simulink model "BatteryModel2RC"  (R2019a)
settings: Solver=VariableStepAuto  StartTime=0.0  StopTime=2417.4  RelTol=1e-3
undefined symbols (not defined in the file): C1Prime, C2Prime, CapacityAh, DiscIntNeverNeededParam, Em, R0, Rx, SOC_LUT
settings Model: Creator=danis  LastModifiedBy=danis

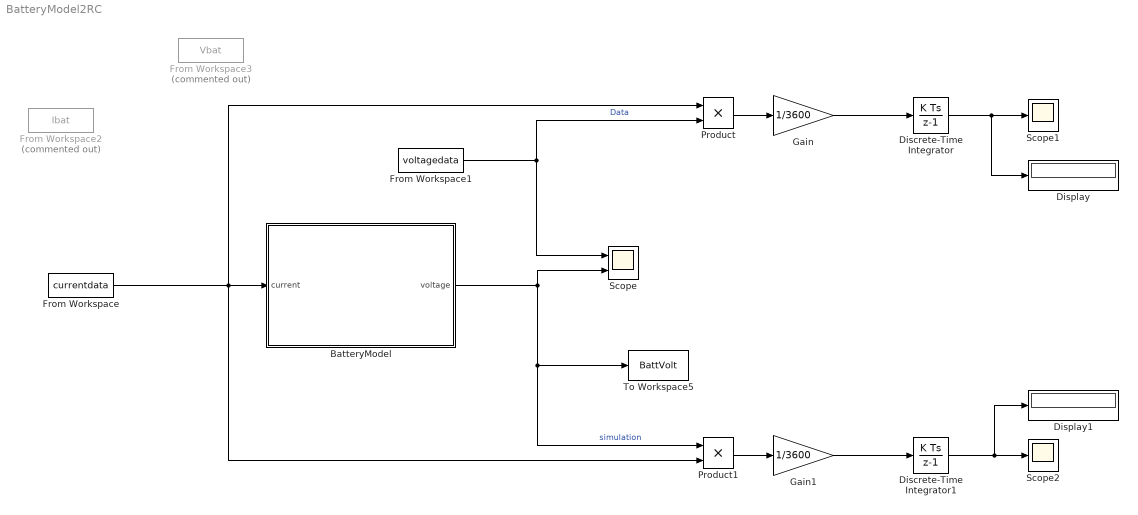
== system BatteryModel2RC ==
  BatteryModel : Subsystem
  Discrete-Time Integrator : DiscreteIntegrator  SampleTime=-1  ICPrevOutput=DiscIntNeverNeededParam  ICPrevScaledInput=DiscIntNeverNeededParam
  Discrete-Time Integrator1 : DiscreteIntegrator  SampleTime=-1  ICPrevOutput=DiscIntNeverNeededParam  ICPrevScaledInput=DiscIntNeverNeededParam
  Display : Display
  Display1 : Display
  From Workspace : FromWorkspace  VariableName=currentdata  SampleTime=0
  From Workspace1 : FromWorkspace  VariableName=voltagedata  SampleTime=0
  From Workspace2 : FromWorkspace  Commented=on  VariableName=Ibat  SampleTime=0.001  Interpolate=off  OutputAfterFinalValue=Cyclic repetition
  From Workspace3 : FromWorkspace  Commented=on  VariableName=Vbat  SampleTime=0.001  Interpolate=off  OutputAfterFinalValue=Cyclic repetition
  Gain : Gain  Gain=1/3600
  Gain1 : Gain  Gain=1/3600
  Product : Product
  Product1 : Product
  Scope : Scope  NumInputPorts=2
  Scope1 : Scope
  Scope2 : Scope
  To Workspace5 : ToWorkspace  VariableName=BattVolt  SampleTime=-1
  wires:
  From Workspace1/1 -> Scope/1, Product/2  "Data"
  BatteryModel/1(voltage) -> Product1/1, To Workspace5/1, Scope/2  "simulation"
  From Workspace/1 -> Product1/2, Product/1, BatteryModel/1(current)
  Product/1 -> Gain/1
  Gain/1 -> Discrete-Time Integrator/1
  Discrete-Time Integrator/1 -> Display/1, Scope1/1
  Discrete-Time Integrator1/1 -> Display1/1, Scope2/1
  Gain1/1 -> Discrete-Time Integrator1/1
  Product1/1 -> Gain1/1

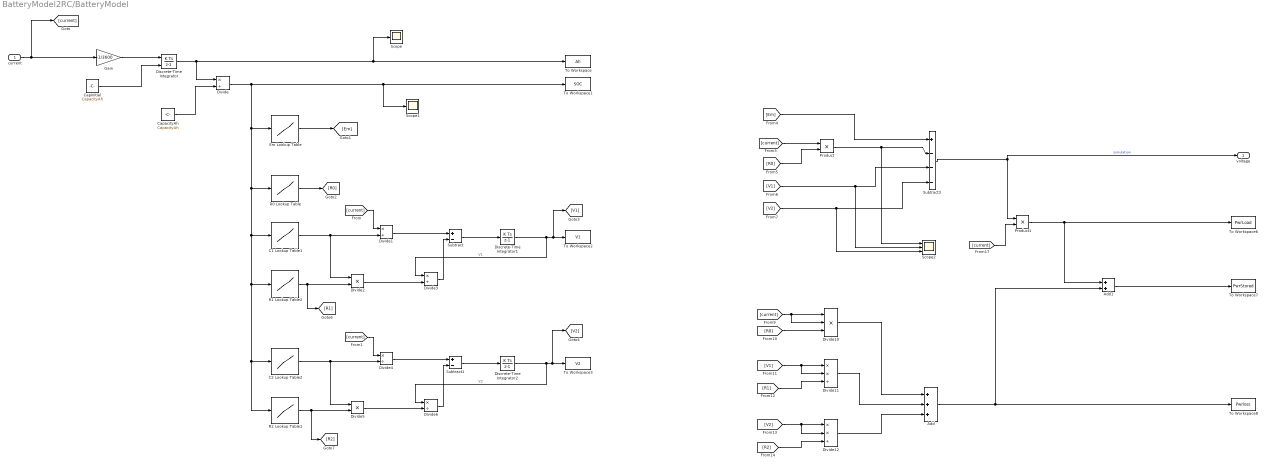
== system BatteryModel2RC/BatteryModel ==
  current : Inport
  Add : Sum  Inputs=+++
  Add1 : Sum
  C1 Lookup Table1 : Lookup_n-D  NumberOfTableDimensions=1  BreakpointsForDimension1=SOC_LUT  Table=C1Prime(1,:)  InternalRulePriority=Speed  RndMeth=Simplest  InputSameDT=on
  C2 Lookup Table2 : Lookup_n-D  NumberOfTableDimensions=1  BreakpointsForDimension1=SOC_LUT  Table=C2Prime(1,:)  InternalRulePriority=Speed  RndMeth=Simplest  InputSameDT=on
  CapInitial : Constant  Value=CapacityAh  SampleTime=0.001
  CapacityAh : Constant  Value=CapacityAh  SampleTime=0.001
  Discrete-Time Integrator : DiscreteIntegrator  InitialConditionSource=external  SampleTime=-1  ICPrevOutput=DiscIntNeverNeededParam  ICPrevScaledInput=DiscIntNeverNeededParam
  Discrete-Time Integrator1 : DiscreteIntegrator  SampleTime=-1  ICPrevOutput=DiscIntNeverNeededParam  ICPrevScaledInput=DiscIntNeverNeededParam
  Discrete-Time Integrator2 : DiscreteIntegrator  SampleTime=-1  ICPrevOutput=DiscIntNeverNeededParam  ICPrevScaledInput=DiscIntNeverNeededParam
  Divide{,1,3..4,6} (5 alike) : Product  Inputs=*/
  Divide10 : Product  Inputs=***
  Divide11 : Product  Inputs=**/
  Divide12 : Product  Inputs=**/
  Divide2 : Product  Inputs=**
  Divide5 : Product  Inputs=**
  Em Lookup Table : Lookup_n-D  NumberOfTableDimensions=1  BreakpointsForDimension1=SOC_LUT  Table=Em  InternalRulePriority=Speed  RndMeth=Simplest  InputSameDT=on
  Gain : Gain  Gain=-1/3600
  Product : Product
  Product1 : Product
  R0 Lookup Table : Lookup_n-D  NumberOfTableDimensions=1  BreakpointsForDimension1=SOC_LUT  Table=R0  InternalRulePriority=Speed  RndMeth=Simplest  InputSameDT=on
  R1 Lookup Table2 : Lookup_n-D  NumberOfTableDimensions=1  BreakpointsForDimension1=SOC_LUT  Table=Rx(1,:)  InternalRulePriority=Speed  RndMeth=Simplest  InputSameDT=on
  R2 Lookup Table1 : Lookup_n-D  NumberOfTableDimensions=1  BreakpointsForDimension1=SOC_LUT  Table=Rx(2,:)  InternalRulePriority=Speed  RndMeth=Simplest  InputSameDT=on
  Scope : Scope
  Scope1 : Scope
  Scope2 : Scope  NumInputPorts=3
  Subtract : Sum  Inputs=+-
  Subtract1 : Sum  Inputs=+-
  Subtract3 : Sum  Inputs=+---
  To Workspace : ToWorkspace  VariableName=Ah  SampleTime=-1
  To Workspace1 : ToWorkspace  VariableName=SOC  SampleTime=-1
  To Workspace2 : ToWorkspace  VariableName=V1  SampleTime=-1
  To Workspace3 : ToWorkspace  VariableName=V2  SampleTime=-1
  To Workspace6 : ToWorkspace  VariableName=PwrLoad  SampleTime=-1
  To Workspace7 : ToWorkspace  VariableName=PwrStored  SampleTime=-1
  To Workspace8 : ToWorkspace  VariableName=Pwrloss  SampleTime=-1
  voltage : Outport
  wires:
  Discrete-Time Integrator2/1 -> Divide6/1, To Workspace3/1, [V2]  "V2"
  Divide4/1 -> Subtract1/1
  [R0] -> Product/2
  Discrete-Time Integrator/1 -> Scope/1, To Workspace/1, Divide/1
  C2 Lookup Table2/1 -> Divide5/1, Divide4/2
  C1 Lookup Table1/1 -> Divide2/1, Divide1/2
  Gain/1 -> Discrete-Time Integrator/1
  [current] -> Product1/2
  Divide3/1 -> Subtract/2
  Divide6/1 -> Subtract1/2
  [Em] -> Subtract3/1
  Divide5/1 -> Divide6/2
  Subtract/1 -> Discrete-Time Integrator1/1
  R2 Lookup Table1/1 -> [R2], Divide5/2
  Divide/1 -> Scope1/1, To Workspace1/1, R2 Lookup Table1/1, C2 Lookup Table2/1, R1 Lookup Table2/1, C1 Lookup Table1/1, R0 Lookup Table/1, Em Lookup Table/1
  Divide2/1 -> Divide3/2
  Divide1/1 -> Subtract/1
  CapacityAh/1 -> Divide/2
  [current] -> Divide10/2, Divide10/1
  Discrete-Time Integrator1/1 -> Divide3/1, To Workspace2/1, [V1]  "V1"
  Divide10/1 -> Add/1
  [V1] -> Divide11/2, Divide11/1
  Subtract1/1 -> Discrete-Time Integrator2/1
  [current] -> Product/1
  [current] -> Divide4/1
  [V2] -> Scope2/3, Subtract3/4
  [R1] -> Divide11/3
  R1 Lookup Table2/1 -> [R1], Divide2/2
  Product/1 -> Scope2/1, Subtract3/2
  Em Lookup Table/1 -> [Em]
  [V1] -> Scope2/2, Subtract3/3
  [R0] -> Divide10/3
  Divide11/1 -> Add/2
  [current] -> Divide1/1
  Divide12/1 -> Add/3
  R0 Lookup Table/1 -> [R0]
  [R2] -> Divide12/3
  Subtract3/1 -> voltage/1, Product1/1  "simulation"
  Add1/1 -> To Workspace7/1
  [V2] -> Divide12/2, Divide12/1
  Add/1 -> To Workspace8/1, Add1/2
  Product1/1 -> To Workspace6/1, Add1/1
  current/1 -> [current], Gain/1
  CapInitial/1 -> Discrete-Time Integrator/2
